simulink model "swingCatchSim"  (R2025a)
settings: Solver=FixedStepAuto  StartTime=0.0  StopTime=20  FixedStep=0.02  RelTol=1e-3
undefined symbols (not defined in the file): K
libraries: slpidlib x4
settings Model: Creator=thinkpad  LastModifiedBy=thinkpad

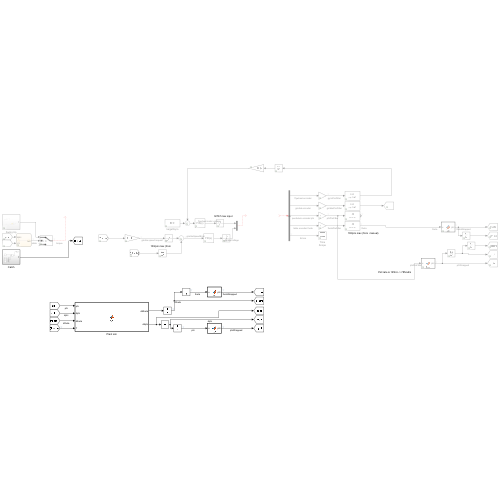
[thumbnail: Simulink's stored preview of the top-level diagram]
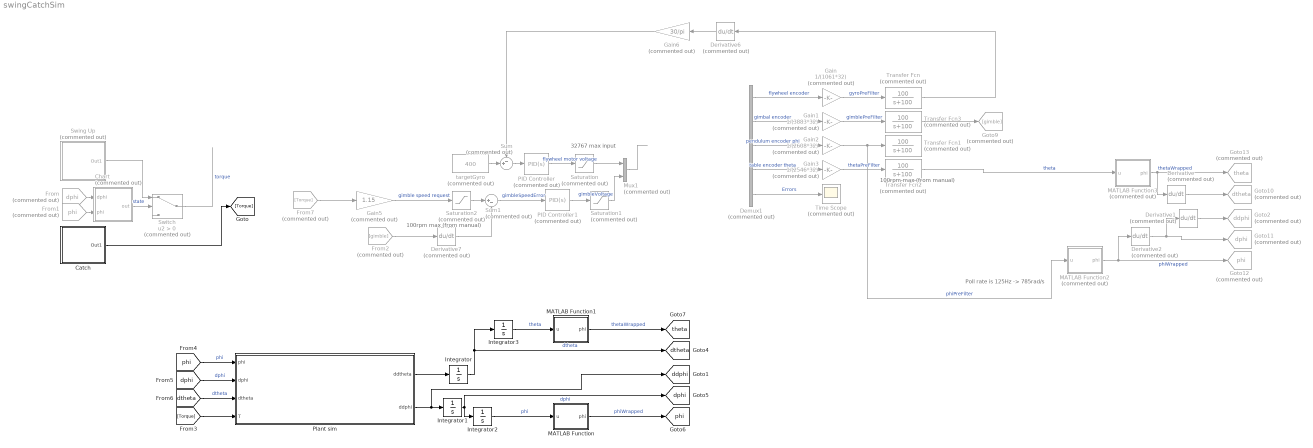
== system swingCatchSim ==
  note: 100rpm max (from manual)
  note: 100rpm max (from manual)
  note: 32767 max input
  note: Poll rate is 125Hz -> 785rad/s
  Catch : Subsystem
  Chart : Stateflow chart  Commented=on  TreatAsAtomicUnit=on
  Demux1 : Demux  Commented=on  Outputs=5
      settings: DisplayOption=none
  Derivative{,1..2,6..7} (5 alike) : Derivative  Commented=on
  From : From  Commented=on  GotoTag=dphi  TagVisibility=global
  From1 : From  Commented=on  GotoTag=phi  TagVisibility=global
  From2 : From  Commented=on  GotoTag=gimble
  From7 : From  Commented=on  GotoTag=Torque
  Gain : Gain  Commented=on  Gain=1/(1061*32)
  Gain1 : Gain  Commented=on  Gain=1/(3883*32)
  Gain2 : Gain  Commented=on  Gain=1/(2608*32)
  Gain3 : Gain  Commented=on  Gain=1/(2546*32)
  Gain5 : Gain  Commented=on  Gain=1.15
  Gain6 : Gain  Commented=on  Gain=30/pi
  Goto10 : Goto  Commented=on  GotoTag=dtheta  TagVisibility=global
  Goto11 : Goto  Commented=on  GotoTag=dphi  TagVisibility=global
  Goto12 : Goto  Commented=on  GotoTag=phi  TagVisibility=global
  Goto13 : Goto  Commented=on  GotoTag=theta  TagVisibility=global
  Goto2 : Goto  Commented=on  GotoTag=ddphi  TagVisibility=global
  Goto9 : Goto  Commented=on  GotoTag=gimble
  Integrator : Integrator
  Integrator1 : Integrator
  Integrator2 : Integrator  InitialCondition=15*pi/180
  Integrator3 : Integrator
  MATLAB Function : MATLAB Function  TreatAsAtomicUnit=on
  MATLAB Function1 : MATLAB Function  TreatAsAtomicUnit=on
  MATLAB Function2 : MATLAB Function  Commented=on  TreatAsAtomicUnit=on
  MATLAB Function3 : MATLAB Function  Commented=on  TreatAsAtomicUnit=on
  Mux1 : Mux  Commented=on  Inputs=2
  PID Controller : slpidlib/PID Controller  Commented=on  Controller=PID  Form=Parallel  TimeDomain=Continuous-time  UseExternalTs=off  SampleTime=-1  IntegratorMethod=Forward Euler  FilterMethod=Forward Euler  ControllerParametersSource=internal  P=4000  I=2  UseKiTs=off  D=1  UseExternalDerivativeSource=off  N=100  UseFilter=on  TunerSelectOption=Transfer Function Based (PID Tuner App)  InitialConditionSource=internal  InitialConditionForIntegrator=0  InitialConditionForFilter=0  DifferentiatorICPrevScaledInput=0  ExternalReset=none  TrackingMode=off  Kt=1  LimitOutput=off  SatLimitsSource=internal  UpperSaturationLimit=32000  LowerSaturationLimit=-32000  LinearizeAsGain=on  AntiWindupMode=none  Kb=1  LimitIntegrator=off  UpperIntegratorSaturationLimit=inf  LowerIntegratorSaturationLimit=-inf  POutMin=[]  POutMax=[]  IOutMin=[]  IOutMax=[]  DOutMin=[]  DOutMax=[]  NOutMin=[]  NOutMax=[]  SumOutMin=[]  SumOutMax=[]  SaturationOutMin=[]  SaturationOutMax=[]  PParamMin=[]  PParamMax=[]  IParamMin=[]  IParamMax=[]  DParamMin=[]  DParamMax=[]  NParamMin=[]  NParamMax=[]  KbParamMin=[]  KbParamMax=[]  KtParamMin=[]  KtParamMax=[]  KbOutMin=[]  KbOutMax=[]  KtOutMin=[]  KtOutMax=[]  IntegratorOutMin=[]  IntegratorOutMax=[]  FilterOutMin=[]  FilterOutMax=[]  SumI1OutMin=[]  SumI1OutMax=[]  SumI2OutMin=[]  SumI2OutMax=[]  SumI3OutMin=[]  SumI3OutMax=[]  SumI4OutMin=[]  SumI4OutMax=[]  SumDOutMin=[]  SumDOutMax=[]  DifferentiatorOutMin=[]  DifferentiatorOutMax=[]  FilterDiffOutCoefMin=[]  FilterDiffOutCoefMax=[]  ReciprocalOutMin=[]  ReciprocalOutMax=[]  SumDenOutMin=[]  SumDenOutMax=[]  SumNumOutMin=[]  SumNumOutMax=[]  DivideOutMin=[]  DivideOutMax=[]  UdiffTsProdOutMin=[]  UdiffTsProdOutMax=[]  NTsProdOutMin=[]  NTsProdOutMax=[]  UintegralTsProdOutMin=[]  UintegralTsProdOutMax=[]  UngainTsProdOutMin=[]  UngainTsProdOutMax=[]  ClampingZeroOutDataTypeStr=Inherit: Inherit via back propagation  ClampingZeroOutMin=[]  ClampingZeroOutMax=[]  FilterDenConstantOutDataTypeStr=Inherit: Inherit via back propagation  FilterDenConstantOutMin=[]  FilterDenConstantOutMax=[]  PCopyOutDataTypeStr=Inherit: Inherit via back propagation  PCopyOutMin=[]  PCopyOutMax=[]  NCopyOutDataTypeStr=Inherit: Inherit via back propagation  NCopyOutMin=[]  NCopyOutMax=[]  IntegratorContinuousStateAttributes=''  IntegratorStateMustResolveToSignalObject=off  IntegratorRTWStateStorageClass=Auto  FilterContinuousStateAttributes=''  FilterStateMustResolveToSignalObject=off  FilterRTWStateStorageClass=Auto  ParallelPVariant=InternalParameters  IdealPVariant=Disabled  IVariant=InternalParameters  DVariant=InternalParameters  IntegratorVariant=Continuous  SatVariant=Disabled  AWVariant=Passthrough  PCopyVariant=Disabled  TRVariant=Disabled  FdbkBlocksVariant=Forward  IdealPFdbkVariant=Disabled  SatFdbkVariant=Disabled  DerivativeFilterVariant=ContFilter  NVariant=InternalParameters  NCopyVariant=Disabled  FilterICVariant=InternalICsFilter  IntegratorICVariant=InternalICs  ExternalResetVariant=Disabled  TRSumVariant=Passthrough  SumFdbkVariant=Disabled  SumVariant=Sum_PID  TsampFilterVariant=InternalTs  TsampNgainVariant=Passthrough  TsampIntegralVariant=Disabled_SignalSpec  ExternalSaturationOutDataTypeStr=Inherit: Same as second input  DerivativeSourceVariant=ErrorSignal  PreIntVariant=InternalPreInt
  PID Controller1 : slpidlib/PID Controller  Commented=on  Controller=PID  Form=Parallel  TimeDomain=Continuous-time  UseExternalTs=off  SampleTime=-1  IntegratorMethod=Forward Euler  FilterMethod=Forward Euler  ControllerParametersSource=internal  P=8000  I=500  UseKiTs=off  D=0  UseExternalDerivativeSource=off  N=100  UseFilter=on  TunerSelectOption=Transfer Function Based (PID Tuner App)  InitialConditionSource=internal  InitialConditionForIntegrator=0  InitialConditionForFilter=0  DifferentiatorICPrevScaledInput=0  ExternalReset=none  TrackingMode=off  Kt=1  LimitOutput=off  SatLimitsSource=internal  UpperSaturationLimit=23500  LowerSaturationLimit=-23500  LinearizeAsGain=on  AntiWindupMode=none  Kb=1  LimitIntegrator=off  UpperIntegratorSaturationLimit=inf  LowerIntegratorSaturationLimit=-inf  POutMin=[]  POutMax=[]  IOutMin=[]  IOutMax=[]  DOutMin=[]  DOutMax=[]  NOutMin=[]  NOutMax=[]  SumOutMin=[]  SumOutMax=[]  SaturationOutMin=[]  SaturationOutMax=[]  PParamMin=[]  PParamMax=[]  IParamMin=[]  IParamMax=[]  DParamMin=[]  DParamMax=[]  NParamMin=[]  NParamMax=[]  KbParamMin=[]  KbParamMax=[]  KtParamMin=[]  KtParamMax=[]  KbOutMin=[]  KbOutMax=[]  KtOutMin=[]  KtOutMax=[]  IntegratorOutMin=[]  IntegratorOutMax=[]  FilterOutMin=[]  FilterOutMax=[]  SumI1OutMin=[]  SumI1OutMax=[]  SumI2OutMin=[]  SumI2OutMax=[]  SumI3OutMin=[]  SumI3OutMax=[]  SumI4OutMin=[]  SumI4OutMax=[]  SumDOutMin=[]  SumDOutMax=[]  DifferentiatorOutMin=[]  DifferentiatorOutMax=[]  FilterDiffOutCoefMin=[]  FilterDiffOutCoefMax=[]  ReciprocalOutMin=[]  ReciprocalOutMax=[]  SumDenOutMin=[]  SumDenOutMax=[]  SumNumOutMin=[]  SumNumOutMax=[]  DivideOutMin=[]  DivideOutMax=[]  UdiffTsProdOutMin=[]  UdiffTsProdOutMax=[]  NTsProdOutMin=[]  NTsProdOutMax=[]  UintegralTsProdOutMin=[]  UintegralTsProdOutMax=[]  UngainTsProdOutMin=[]  UngainTsProdOutMax=[]  ClampingZeroOutDataTypeStr=Inherit: Inherit via back propagation  ClampingZeroOutMin=[]  ClampingZeroOutMax=[]  FilterDenConstantOutDataTypeStr=Inherit: Inherit via back propagation  FilterDenConstantOutMin=[]  FilterDenConstantOutMax=[]  PCopyOutDataTypeStr=Inherit: Inherit via back propagation  PCopyOutMin=[]  PCopyOutMax=[]  NCopyOutDataTypeStr=Inherit: Inherit via back propagation  NCopyOutMin=[]  NCopyOutMax=[]  IntegratorContinuousStateAttributes=''  IntegratorStateMustResolveToSignalObject=off  IntegratorRTWStateStorageClass=Auto  FilterContinuousStateAttributes=''  FilterStateMustResolveToSignalObject=off  FilterRTWStateStorageClass=Auto  ParallelPVariant=InternalParameters  IdealPVariant=Disabled  IVariant=InternalParameters  DVariant=InternalParameters  IntegratorVariant=Continuous  SatVariant=Disabled  AWVariant=Passthrough  PCopyVariant=Disabled  TRVariant=Disabled  FdbkBlocksVariant=Forward  IdealPFdbkVariant=Disabled  SatFdbkVariant=Disabled  DerivativeFilterVariant=ContFilter  NVariant=InternalParameters  NCopyVariant=Disabled  FilterICVariant=InternalICsFilter  IntegratorICVariant=InternalICs  ExternalResetVariant=Disabled  TRSumVariant=Passthrough  SumFdbkVariant=Disabled  SumVariant=Sum_PID  TsampFilterVariant=InternalTs  TsampNgainVariant=Passthrough  TsampIntegralVariant=Disabled_SignalSpec  ExternalSaturationOutDataTypeStr=Inherit: Same as second input  DerivativeSourceVariant=ErrorSignal  PreIntVariant=InternalPreInt
  Plant sim : MATLAB Function  TreatAsAtomicUnit=on
  Saturation : Saturate  Commented=on  UpperLimit=30000  LowerLimit=-30000
  Saturation1 : Saturate  Commented=on  UpperLimit=30000  LowerLimit=-30000
  Saturation2 : Saturate  Commented=on  UpperLimit=10  LowerLimit=-10
  Sum : Sum  Commented=on  Inputs=-+|
  Sum1 : Sum  Commented=on  Inputs=|+-
  Swing Up : Subsystem  Commented=on
  Switch : Switch  Commented=on  Criteria=u2 > Threshold  SaturateOnIntegerOverflow=off  InputSameDT=off
  Time Scope : Scope  Commented=on
      settings: TimeUnits=Metric (based on Time Span)  ActiveDisplayYMinimum=-1  ActiveDisplayYMaximum=1  YLabel=Amplitude
  Transfer Fcn{,1..3} (4 alike) : TransferFcn  Commented=on  Numerator=[100]  Denominator=[1 100]
  targetGyro : Constant  Commented=on  Value=400
  tag scope: ddphi=global, dphi=global, dtheta=global, phi=global, theta=global
  wires:
  Integrator1/1 -> [dphi], Integrator2/1  "dphi"
  Integrator2/1 -> MATLAB Function/1(u)  "phi"
  [Torque] -> Plant sim/4(T)
  [phi] -> Plant sim/1(phi)  "phi"
  Integrator3/1 -> MATLAB Function1/1(u)  "theta"
  Plant sim/1(ddtheta) -> Integrator/1
  [dtheta] -> Plant sim/3(dtheta)  "dtheta"
  [dphi] -> Plant sim/2(dphi)  "dphi"
  Integrator/1 -> Integrator3/1, [dtheta]  "dtheta"
  Plant sim/2(ddphi) -> [ddphi], Integrator1/1
  Chart/1(out) -> Switch/2  "state"
  Swing Up/1(Out1) -> Switch/1
  Catch/1(Out1) -> [Torque]
  From/1 -> Chart/1(dphi)
  From1/1 -> Chart/2(phi)
  Switch/1 -> ?  "torque"
  MATLAB Function/1(phi) -> [phi]  "phiWrapped"
  MATLAB Function1/1(phi) -> [theta]  "thetaWrapped"
  Demux1/5 -> Time Scope/1  "Errors"
  ? -> Demux1/1
  targetGyro/1 -> Sum/2
  From2/1 -> Derivative7/1
  Demux1/4 -> Gain3/1  "table encoder theta"
  Sum1/1 -> PID Controller1/1  "gimbleSpeedError"
  Demux1/3 -> Gain2/1  "pendulum encoder phi"
  Saturation/1 -> Mux1/1
  Sum/1 -> PID Controller/1
  PID Controller1/1 -> Saturation1/1
  Mux1/1 -> ?
  PID Controller/1 -> Saturation/1  "flywheel motor voltage"
  Transfer Fcn/1 -> Derivative6/1
  Saturation2/1 -> Sum1/1
  Gain5/1 -> Saturation2/1  "gimble speed request"
  Saturation1/1 -> Mux1/2  "gimbleVoltage"
  Demux1/1 -> Gain/1  "flywheel encoder"
  Derivative7/1 -> Sum1/2
  Demux1/2 -> Gain1/1  "gimbal encoder"
  Gain2/1 -> MATLAB Function2/1(u), Transfer Fcn1/1  "phiPreFilter"
  Gain1/1 -> Transfer Fcn3/1  "gimblePreFilter"
  Derivative6/1 -> Gain6/1
  Gain3/1 -> Transfer Fcn2/1  "thetaPreFilter"
  Gain/1 -> Transfer Fcn/1  "gyroPreFilter"
  Gain6/1 -> Sum/1
  Transfer Fcn3/1 -> Goto9/1
  From7/1 -> Gain5/1
  MATLAB Function3/1(phi) -> Derivative/1, Goto13/1  "thetaWrapped"
  Transfer Fcn2/1 -> MATLAB Function3/1(u)  "theta"
  MATLAB Function2/1(phi) -> Derivative2/1, Goto12/1  "phiWrapped"
  Derivative/1 -> Goto10/1
  Derivative2/1 -> Derivative1/1, Goto11/1
  Derivative1/1 -> Goto2/1

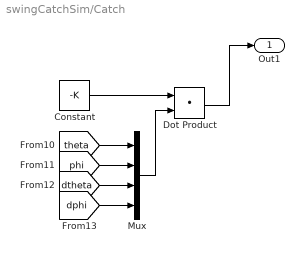
== system swingCatchSim/Catch ==
  Constant : Constant  Value=-K
  Dot Product : DotProduct  OutDataTypeStr=Inherit: Inherit via internal rule
  Mux : Mux
  Out1 : Outport
  wires:
  Constant/1 -> Dot Product/1
  [dtheta] -> Mux/3
  Mux/1 -> Dot Product/2
  Dot Product/1 -> Out1/1
  [theta] -> Mux/1
  [phi] -> Mux/2
  [dphi] -> Mux/4

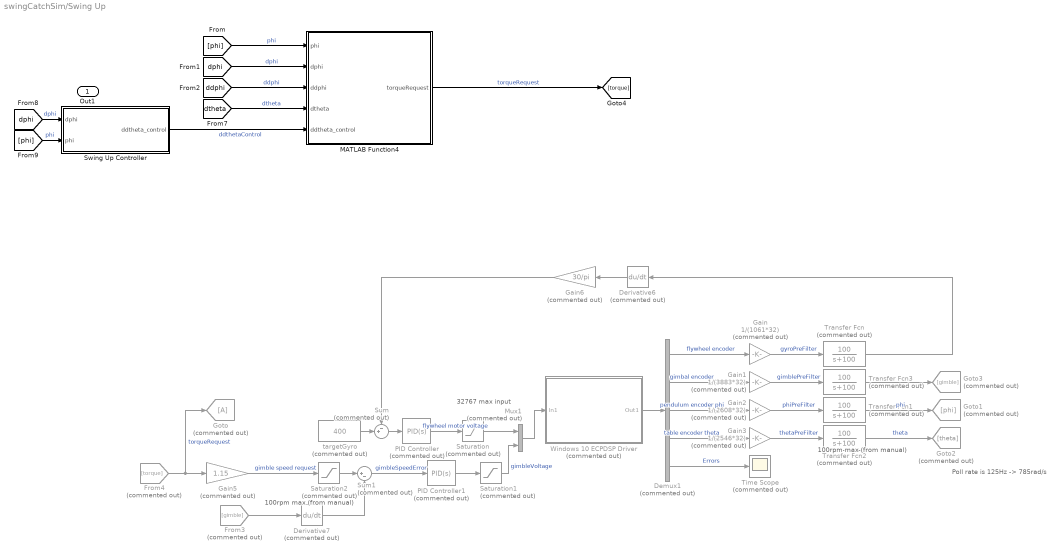
== system swingCatchSim/Swing Up ==
  note: 100rpm max (from manual)
  note: 100rpm max (from manual)
  note: 32767 max input
  note: Poll rate is 125Hz -> 785rad/s
  Demux1 : Demux  Commented=on  Outputs=5
      settings: DisplayOption=none
  Derivative6 : Derivative  Commented=on
  Derivative7 : Derivative  Commented=on
  From3 : From  Commented=on  GotoTag=gimble
  From4 : From  Commented=on  GotoTag=torque
  Gain : Gain  Commented=on  Gain=1/(1061*32)
  Gain1 : Gain  Commented=on  Gain=1/(3883*32)
  Gain2 : Gain  Commented=on  Gain=1/(2608*32)
  Gain3 : Gain  Commented=on  Gain=1/(2546*32)
  Gain5 : Gain  Commented=on  Gain=1.15
  Gain6 : Gain  Commented=on  Gain=30/pi
  Goto : Goto  Commented=on
  Goto1 : Goto  Commented=on  GotoTag=phi
  Goto2 : Goto  Commented=on  GotoTag=theta
  Goto3 : Goto  Commented=on  GotoTag=gimble
  MATLAB Function4 : MATLAB Function  TreatAsAtomicUnit=on
  Mux1 : Mux  Commented=on  Inputs=2
  PID Controller : slpidlib/PID Controller  Commented=on  Controller=PID  Form=Parallel  TimeDomain=Continuous-time  UseExternalTs=off  SampleTime=-1  IntegratorMethod=Forward Euler  FilterMethod=Forward Euler  ControllerParametersSource=internal  P=4000  I=2  UseKiTs=off  D=1  UseExternalDerivativeSource=off  N=100  UseFilter=on  TunerSelectOption=Transfer Function Based (PID Tuner App)  InitialConditionSource=internal  InitialConditionForIntegrator=0  InitialConditionForFilter=0  DifferentiatorICPrevScaledInput=0  ExternalReset=none  TrackingMode=off  Kt=1  LimitOutput=off  SatLimitsSource=internal  UpperSaturationLimit=32000  LowerSaturationLimit=-32000  LinearizeAsGain=on  AntiWindupMode=none  Kb=1  LimitIntegrator=off  UpperIntegratorSaturationLimit=inf  LowerIntegratorSaturationLimit=-inf  POutMin=[]  POutMax=[]  IOutMin=[]  IOutMax=[]  DOutMin=[]  DOutMax=[]  NOutMin=[]  NOutMax=[]  SumOutMin=[]  SumOutMax=[]  SaturationOutMin=[]  SaturationOutMax=[]  PParamMin=[]  PParamMax=[]  IParamMin=[]  IParamMax=[]  DParamMin=[]  DParamMax=[]  NParamMin=[]  NParamMax=[]  KbParamMin=[]  KbParamMax=[]  KtParamMin=[]  KtParamMax=[]  KbOutMin=[]  KbOutMax=[]  KtOutMin=[]  KtOutMax=[]  IntegratorOutMin=[]  IntegratorOutMax=[]  FilterOutMin=[]  FilterOutMax=[]  SumI1OutMin=[]  SumI1OutMax=[]  SumI2OutMin=[]  SumI2OutMax=[]  SumI3OutMin=[]  SumI3OutMax=[]  SumI4OutMin=[]  SumI4OutMax=[]  SumDOutMin=[]  SumDOutMax=[]  DifferentiatorOutMin=[]  DifferentiatorOutMax=[]  FilterDiffOutCoefMin=[]  FilterDiffOutCoefMax=[]  ReciprocalOutMin=[]  ReciprocalOutMax=[]  SumDenOutMin=[]  SumDenOutMax=[]  SumNumOutMin=[]  SumNumOutMax=[]  DivideOutMin=[]  DivideOutMax=[]  UdiffTsProdOutMin=[]  UdiffTsProdOutMax=[]  NTsProdOutMin=[]  NTsProdOutMax=[]  UintegralTsProdOutMin=[]  UintegralTsProdOutMax=[]  UngainTsProdOutMin=[]  UngainTsProdOutMax=[]  ClampingZeroOutDataTypeStr=Inherit: Inherit via back propagation  ClampingZeroOutMin=[]  ClampingZeroOutMax=[]  FilterDenConstantOutDataTypeStr=Inherit: Inherit via back propagation  FilterDenConstantOutMin=[]  FilterDenConstantOutMax=[]  PCopyOutDataTypeStr=Inherit: Inherit via back propagation  PCopyOutMin=[]  PCopyOutMax=[]  NCopyOutDataTypeStr=Inherit: Inherit via back propagation  NCopyOutMin=[]  NCopyOutMax=[]  IntegratorContinuousStateAttributes=''  IntegratorStateMustResolveToSignalObject=off  IntegratorRTWStateStorageClass=Auto  FilterContinuousStateAttributes=''  FilterStateMustResolveToSignalObject=off  FilterRTWStateStorageClass=Auto  ParallelPVariant=InternalParameters  IdealPVariant=Disabled  IVariant=InternalParameters  DVariant=InternalParameters  IntegratorVariant=Continuous  SatVariant=Disabled  AWVariant=Passthrough  PCopyVariant=Disabled  TRVariant=Disabled  FdbkBlocksVariant=Forward  IdealPFdbkVariant=Disabled  SatFdbkVariant=Disabled  DerivativeFilterVariant=ContFilter  NVariant=InternalParameters  NCopyVariant=Disabled  FilterICVariant=InternalICsFilter  IntegratorICVariant=InternalICs  ExternalResetVariant=Disabled  TRSumVariant=Passthrough  SumFdbkVariant=Disabled  SumVariant=Sum_PID  TsampFilterVariant=InternalTs  TsampNgainVariant=Passthrough  TsampIntegralVariant=Disabled_SignalSpec  ExternalSaturationOutDataTypeStr=Inherit: Same as second input  DerivativeSourceVariant=ErrorSignal  PreIntVariant=InternalPreInt
  PID Controller1 : slpidlib/PID Controller  Commented=on  Controller=PID  Form=Parallel  TimeDomain=Continuous-time  UseExternalTs=off  SampleTime=-1  IntegratorMethod=Forward Euler  FilterMethod=Forward Euler  ControllerParametersSource=internal  P=8000  I=500  UseKiTs=off  D=0  UseExternalDerivativeSource=off  N=100  UseFilter=on  TunerSelectOption=Transfer Function Based (PID Tuner App)  InitialConditionSource=internal  InitialConditionForIntegrator=0  InitialConditionForFilter=0  DifferentiatorICPrevScaledInput=0  ExternalReset=none  TrackingMode=off  Kt=1  LimitOutput=off  SatLimitsSource=internal  UpperSaturationLimit=23500  LowerSaturationLimit=-23500  LinearizeAsGain=on  AntiWindupMode=none  Kb=1  LimitIntegrator=off  UpperIntegratorSaturationLimit=inf  LowerIntegratorSaturationLimit=-inf  POutMin=[]  POutMax=[]  IOutMin=[]  IOutMax=[]  DOutMin=[]  DOutMax=[]  NOutMin=[]  NOutMax=[]  SumOutMin=[]  SumOutMax=[]  SaturationOutMin=[]  SaturationOutMax=[]  PParamMin=[]  PParamMax=[]  IParamMin=[]  IParamMax=[]  DParamMin=[]  DParamMax=[]  NParamMin=[]  NParamMax=[]  KbParamMin=[]  KbParamMax=[]  KtParamMin=[]  KtParamMax=[]  KbOutMin=[]  KbOutMax=[]  KtOutMin=[]  KtOutMax=[]  IntegratorOutMin=[]  IntegratorOutMax=[]  FilterOutMin=[]  FilterOutMax=[]  SumI1OutMin=[]  SumI1OutMax=[]  SumI2OutMin=[]  SumI2OutMax=[]  SumI3OutMin=[]  SumI3OutMax=[]  SumI4OutMin=[]  SumI4OutMax=[]  SumDOutMin=[]  SumDOutMax=[]  DifferentiatorOutMin=[]  DifferentiatorOutMax=[]  FilterDiffOutCoefMin=[]  FilterDiffOutCoefMax=[]  ReciprocalOutMin=[]  ReciprocalOutMax=[]  SumDenOutMin=[]  SumDenOutMax=[]  SumNumOutMin=[]  SumNumOutMax=[]  DivideOutMin=[]  DivideOutMax=[]  UdiffTsProdOutMin=[]  UdiffTsProdOutMax=[]  NTsProdOutMin=[]  NTsProdOutMax=[]  UintegralTsProdOutMin=[]  UintegralTsProdOutMax=[]  UngainTsProdOutMin=[]  UngainTsProdOutMax=[]  ClampingZeroOutDataTypeStr=Inherit: Inherit via back propagation  ClampingZeroOutMin=[]  ClampingZeroOutMax=[]  FilterDenConstantOutDataTypeStr=Inherit: Inherit via back propagation  FilterDenConstantOutMin=[]  FilterDenConstantOutMax=[]  PCopyOutDataTypeStr=Inherit: Inherit via back propagation  PCopyOutMin=[]  PCopyOutMax=[]  NCopyOutDataTypeStr=Inherit: Inherit via back propagation  NCopyOutMin=[]  NCopyOutMax=[]  IntegratorContinuousStateAttributes=''  IntegratorStateMustResolveToSignalObject=off  IntegratorRTWStateStorageClass=Auto  FilterContinuousStateAttributes=''  FilterStateMustResolveToSignalObject=off  FilterRTWStateStorageClass=Auto  ParallelPVariant=InternalParameters  IdealPVariant=Disabled  IVariant=InternalParameters  DVariant=InternalParameters  IntegratorVariant=Continuous  SatVariant=Disabled  AWVariant=Passthrough  PCopyVariant=Disabled  TRVariant=Disabled  FdbkBlocksVariant=Forward  IdealPFdbkVariant=Disabled  SatFdbkVariant=Disabled  DerivativeFilterVariant=ContFilter  NVariant=InternalParameters  NCopyVariant=Disabled  FilterICVariant=InternalICsFilter  IntegratorICVariant=InternalICs  ExternalResetVariant=Disabled  TRSumVariant=Passthrough  SumFdbkVariant=Disabled  SumVariant=Sum_PID  TsampFilterVariant=InternalTs  TsampNgainVariant=Passthrough  TsampIntegralVariant=Disabled_SignalSpec  ExternalSaturationOutDataTypeStr=Inherit: Same as second input  DerivativeSourceVariant=ErrorSignal  PreIntVariant=InternalPreInt
  Saturation : Saturate  Commented=on  UpperLimit=30000  LowerLimit=-30000
  Saturation1 : Saturate  Commented=on  UpperLimit=30000  LowerLimit=-30000
  Saturation2 : Saturate  Commented=on  UpperLimit=10  LowerLimit=-10
  Sum : Sum  Commented=on  Inputs=-+|
  Sum1 : Sum  Commented=on  Inputs=|+-
  Swing Up Controller : MATLAB Function  TreatAsAtomicUnit=on
  Time Scope : Scope  Commented=on
      settings: TimeUnits=Metric (based on Time Span)  ActiveDisplayYMinimum=-1  ActiveDisplayYMaximum=1  YLabel=Amplitude  DataLoggingVariableName=ScopeData3
  Transfer Fcn{,1..3} (4 alike) : TransferFcn  Commented=on  Numerator=[100]  Denominator=[1 100]
  Windows 10 ECPDSP Driver : Subsystem  Commented=on  mask{BaseAddr='0x3F00', STime=0.008, TimeOutPer=500, HWAccess=on}
      mask prompts: BaseAddr "Base I/O Address"; STime "Sample Time (Sec)"; TimeOutPer "Timeout Period (500 ~ 2000)"; HWAccess "Hardware Access"
      mask Display: color('black');disp('ECPDSP Driver\n upto\n 4 Encs(ADC Channels)\n and 2 Dacs')
  targetGyro : Constant  Commented=on  Value=400
  Out1 : Outport
  wires:
  [ddphi] -> MATLAB Function4/3(ddphi)  "ddphi"
  [dtheta] -> MATLAB Function4/4(dtheta)  "dtheta"
  [dphi] -> MATLAB Function4/2(dphi)  "dphi"
  Swing Up Controller/1(ddtheta_control) -> MATLAB Function4/5(ddtheta_control)  "ddthetaControl"
  [phi] -> Swing Up Controller/2(phi)  "phi"
  [phi] -> MATLAB Function4/1(phi)  "phi"
  [dphi] -> Swing Up Controller/1(dphi)  "dphi"
  MATLAB Function4/1(torqueRequest) -> [torque]  "torqueRequest"
  Saturation1/1 -> Mux1/2  "gimbleVoltage"
  Demux1/5 -> Time Scope/1  "Errors"
  Windows 10 ECPDSP Driver/1(Out1) -> Demux1/1
  Transfer Fcn1/1 -> Goto1/1  "phi"
  targetGyro/1 -> Sum/2
  From3/1 -> Derivative7/1
  Demux1/4 -> Gain3/1  "table encoder theta"
  Sum1/1 -> PID Controller1/1  "gimbleSpeedError"
  Transfer Fcn2/1 -> Goto2/1  "theta"
  Demux1/3 -> Gain2/1  "pendulum encoder phi"
  Saturation/1 -> Mux1/1
  Sum/1 -> PID Controller/1
  PID Controller1/1 -> Saturation1/1
  Mux1/1 -> Windows 10 ECPDSP Driver/1(In1)
  PID Controller/1 -> Saturation/1  "flywheel motor voltage"
  Transfer Fcn/1 -> Derivative6/1
  Saturation2/1 -> Sum1/1
  Gain5/1 -> Saturation2/1  "gimble speed request"
  Demux1/2 -> Gain1/1  "gimbal encoder"
  From4/1 -> Goto/1, Gain5/1  "torqueRequest"
  Gain2/1 -> Transfer Fcn1/1  "phiPreFilter"
  Demux1/1 -> Gain/1  "flywheel encoder"
  Derivative7/1 -> Sum1/2
  Gain3/1 -> Transfer Fcn2/1  "thetaPreFilter"
  Gain1/1 -> Transfer Fcn3/1  "gimblePreFilter"
  Derivative6/1 -> Gain6/1
  Gain/1 -> Transfer Fcn/1  "gyroPreFilter"
  Gain6/1 -> Sum/1
  Transfer Fcn3/1 -> Goto3/1

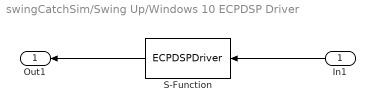
== system swingCatchSim/Swing Up/Windows 10 ECPDSP Driver ==
  In1 : Inport
  S-Function : S-Function  FunctionName=ECPDSPDriver  Parameters=BaseAddr,STime,TimeOutPer,HWAccess  SFunctionDeploymentMode=off  EnableBusSupport=off
  Out1 : Outport
  wires:
  In1/1 -> S-Function/1
  S-Function/1 -> Out1/1

== matlab function swingCatchSim/MATLAB Function ==
  data: u input; phi output
function phi = fcn(u)

phi = wrapToPi(u);

== matlab function swingCatchSim/Plant sim ==
  data: phi input; ddtheta output; dphi input; dtheta input; T input; ddphi output
function [ddtheta, ddphi] = fcn(phi, dphi, dtheta, T)

R = 0.3700
l = 0.2698
r = 0; %reduced into J1_bar
M = 0; %reduced into J1_bar
g = 9.81;
c1 = 1; %friction of base
c2 = 0; %friction of pivot

J =  0.1530 % J1_bar J - inertia of the table
Iyy = 5.5625e-05 %Jy 
I = 0.0131%Jz_bar%  I - inertia of the pendulum
m =     0.1580


ddphi = -(c2*dphi - 0.5000*Iyy*dtheta^2*sin(2*phi) + g*l*m*sin(phi) - 0.5000*dtheta^2*l^2*m*sin(2*phi) + (R*l*m*cos(phi)*(R*m*sin(phi)*dphi^2*l + dtheta*m*sin(2*phi)*dphi*l^2 + Iyy*dtheta*sin(2*phi)*dphi - T + c1*dtheta))/(m*R^2 - m*l^2*cos(phi)^2 + m*l^2 - Iyy*cos(phi)^2 + Iyy + J))/(I + l^2*m - (R^2*l^2*m^2*cos(phi)^2)/(m*R^2 - m*l^2*cos(phi)^2 + m*l^2 - Iyy*cos(phi)^2 + Iyy + J))

ddtheta = -(R*m*sin(phi)*dphi^2*l + dtheta*m*sin(2*phi)*dphi*l^2 + Iyy*dtheta*sin(2*phi)*dphi - R*ddphi*m*cos(phi)*l - T + c1*dtheta)/(m*R^2 - m*l^2*cos(phi)^2 + m*l^2 - Iyy*cos(phi)^2 + Iyy + J);

== stateflow chart swingCatchSim/Chart ==
  state swingUp
    out = 1
  state catch
    out = 0
  (default) -> swingUp
  swingUp -> catch : [abs(phi) < (0.4) && abs(dphi) <=0.4]
  catch -> swingUp : [abs(phi)>12*pi/180]
  data: dphi input; phi input; out output

== matlab function swingCatchSim/Swing Up/Swing Up Controller ==
  data: dphi input; phi input; ddtheta_control output
function ddtheta_control = fcn(dphi, phi)
R = 0.3700;
l = 0.2698;
r = 0; %reduced into J1_bar
M = 0; %reduced into J1_bar
g = 9.81;
c1 = 1; %friction of base
c2 = 0; %friction of pivot

J =  0.1530 % J1_bar J - inertia of the table
Iyy = 5.5625e-05 %Jy 
I = 0.0131%Jz_bar%  I - inertia of the pendulum
m =     0.1580


k = 1
% E = 0.5*I*dphi^2+m*g*l*(cos(phi)-1);
E = 0.5*I*dphi^2 + m*g*l*(cos-1);
ddtheta_control = -((0.5*sin(phi)*(m*l^2+Ixx-Iyy)*dtheta^2)+(k*dphi*cos(phi)))/(m*l*R);

== matlab function swingCatchSim/Swing Up/MATLAB Function4 ==
  data: phi input; dphi input; ddphi input; dtheta input; torqueRequest output; ddtheta_control input
function torqueRequest = fcn(phi, dphi, ddphi,dtheta, ddtheta_control)
R = 0.3700
l = 0.2698
r = 0; %reduced into J1_bar
M = 0; %reduced into J1_bar
g = 9.81;
c1 = 1; %friction of base
c2 = 0; %friction of pivot

J =  0.1530 % J1_bar J - inertia of the table
Iyy = 5.5625e-05 %Jy 
I = 0.0131%Jz_bar%  I - inertia of the pendulum
m =     0.1580


torqueRequest = Iyy*ddtheta_control + J*ddtheta_control + c1*dtheta + ddtheta_control*m*R^2 + ddtheta_control*m*l^2 - Iyy*ddtheta_control*cos(phi)^2 + Iyy*dtheta*sin(2*phi)*dphi - ddtheta_control*m*l^2*cos(phi)^2 + m*sin(phi)*R*dphi^2*l + dtheta*m*sin(2*phi)*dphi*l^2 - ddphi*m*R*l*cos(phi)

== matlab function swingCatchSim/MATLAB Function1 ==
  data: u input; phi output
function phi = fcn(u)

phi = wrapToPi(u);

== matlab function swingCatchSim/MATLAB Function2 ==
  data: u input; phi output
function phi = fcn(u)

phi = wrapToPi(u);

== matlab function swingCatchSim/MATLAB Function3 ==
  data: u input; phi output
function phi = fcn(u)

phi = wrapToPi(u);
